simulink model "voltage_test"  (R2026a)
settings: Solver=VariableStepAuto  StopTime=inf
settings Model: Creator=user  LastModifiedBy=user

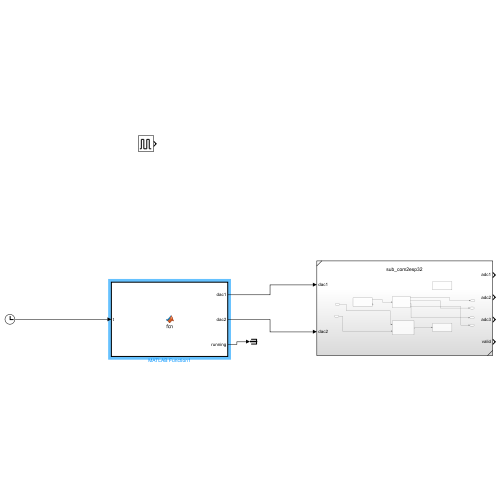
[thumbnail: Simulink's stored preview of the top-level diagram]
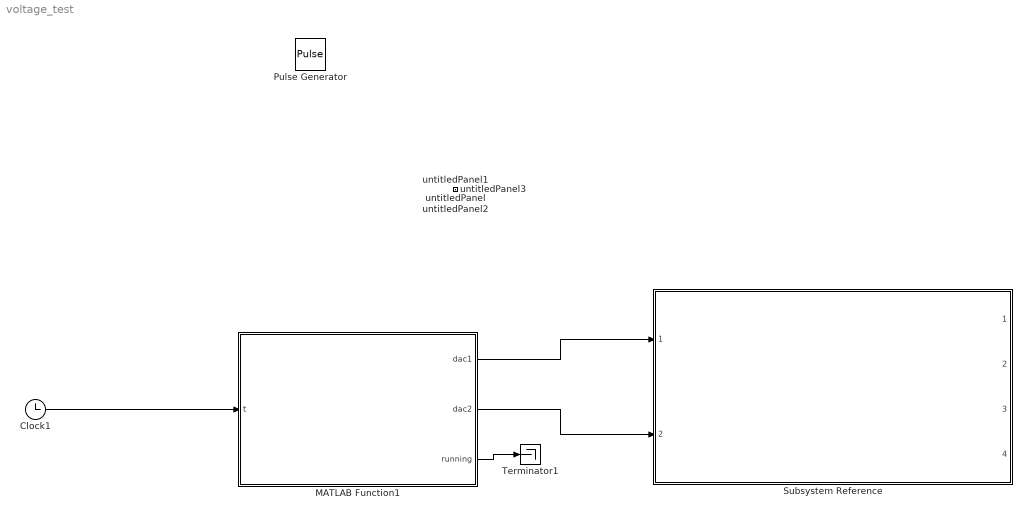
== system voltage_test ==
  Clock1 : Clock
  MATLAB Function1 : MATLAB Function  TreatAsAtomicUnit=on
  Pulse Generator : DiscretePulseGenerator  PulseType=Time based  Period=12  PulseWidth=20
  Subsystem Reference : Subsystem  ReferencedSubsystem=sub_com2esp32
  Terminator1 : Terminator
  untitledPanel : Subsystem  Tag=HiddenForWebPanel  IsWebBlockPanel=on
  untitledPanel1 : Subsystem  Tag=HiddenForWebPanel  IsWebBlockPanel=on
  untitledPanel2 : Subsystem  Tag=HiddenForWebPanel  IsWebBlockPanel=on
  untitledPanel3 : Subsystem  Tag=HiddenForWebPanel  IsWebBlockPanel=on
  wires:
  MATLAB Function1/1(dac1) -> Subsystem Reference/1
  MATLAB Function1/3(running) -> Terminator1/1
  MATLAB Function1/2(dac2) -> Subsystem Reference/2
  Clock1/1 -> MATLAB Function1/1(t)

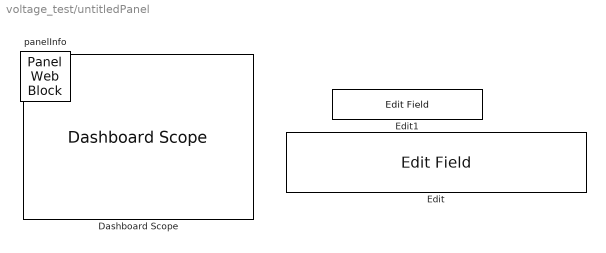
== system voltage_test/untitledPanel ==
  Dashboard Scope : DashboardScope  Tag=HiddenForWebPanel  PanelInfo="{\"height\":195,\"left\":22,\"panelId\":\"panelId-0a8f6d05-5e0e-4052-8464-4cdde78ccbfe\",\"top\":22,\"type\":\"panelChild\",\"version\":\"2019b\",\"width\":271,\"zIndex\":1500002}"  FontColor=[0.0, 0.0, 0.0]
  Edit : EditField  Tag=HiddenForWebPanel  PanelInfo="{\"height\":25,\"left\":322,\"panelId\":\"panelId-0a8f6d05-5e0e-4052-8464-4cdde78ccbfe\",\"top\":100,\"type\":\"panelChild\",\"version\":\"2019b\",\"width\":181,\"zIndex\":1500006}"  LabelPosition=Hide  ShowInitialText=on  Alignment=Center
  Edit1 : EditField  Tag=HiddenForWebPanel  PanelInfo="{\"height\":30,\"left\":327,\"panelId\":\"panelId-0a8f6d05-5e0e-4052-8464-4cdde78ccbfe\",\"top\":53,\"type\":\"panelChild\",\"version\":\"2019b\",\"width\":150,\"zIndex\":1500004}"  LabelPosition=Hide  ShowInitialText=on  Alignment=Center
  panelInfo : PanelWebBlock  Tag=HiddenForWebPanel  PanelInfo="{\"compacted\":false,\"height\":362,\"isActiveTab\":false,\"left\":183,\"name\":\"Panel\",\"panelId\":\"panelId-0a8f6d05-5e0e-4052-8464-4cdde78ccbfe\",\"popoutData\":{\"height\":495,\"left\":546,\"maximized\":false,\"top\":827,\"width\":618},\"popoutMode\":\"windowHidden\",\"tabIndex\":0,\"tabbedSetId\":\"tabbedSet4972758365\",\"top\":737,\"type\":\"panel\",\"version\":\"2019b\",\"visible\":false,\"width\":602,\"zIndex\":1500002}"  PanelSnapshot=<binary blob, 20028 chars, not shown>

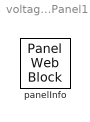
== system voltage_test/untitledPanel1 ==
  panelInfo : PanelWebBlock  Tag=HiddenForWebPanel  PanelInfo="{\"compacted\":false,\"height\":362,\"isActiveTab\":true,\"left\":183,\"name\":\"Panel1\",\"panelId\":\"panelId-b2ee2f41-7720-49f1-b51a-3062c351f597\",\"popoutData\":{\"height\":495,\"left\":546,\"maximized\":false,\"top\":827,\"width\":618},\"popoutMode\":\"windowHidden\",\"tabIndex\":1,\"tabbedSetId\":\"tabbedSet4972758365\",\"top\":737,\"type\":\"panel\",\"version\":\"2019b\",\"visible\":true,\"width\":602,\"zIndex\":1500004}"

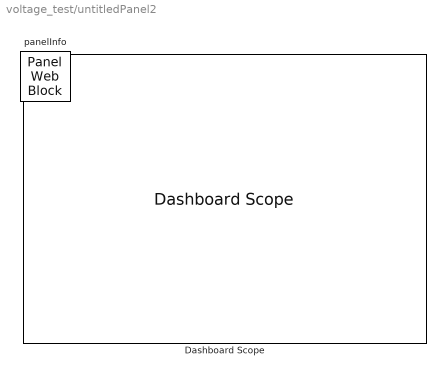
== system voltage_test/untitledPanel2 ==
  Dashboard Scope : DashboardScope  Tag=HiddenForWebPanel  PanelInfo="{\"height\":289,\"left\":18,\"panelId\":\"panelId-8ba459e9-7eb9-43d1-9a8b-2b7bff5a2d5c\",\"top\":18,\"type\":\"panelChild\",\"version\":\"2019b\",\"width\":403,\"zIndex\":1500002}"  FontColor=[0.0, 0.0, 0.0]
  panelInfo : PanelWebBlock  Tag=HiddenForWebPanel  PanelInfo="{\"compacted\":false,\"height\":329,\"isActiveTab\":true,\"left\":1320,\"name\":\"Panel2\",\"panelId\":\"panelId-8ba459e9-7eb9-43d1-9a8b-2b7bff5a2d5c\",\"popoutData\":{\"height\":440,\"left\":1683,\"maximized\":false,\"top\":822,\"width\":459},\"popoutMode\":\"windowHidden\",\"tabIndex\":0,\"tabbedSetId\":\"tabbedSet1724704130\",\"top\":710,\"type\":\"panel\",\"version\":\"2019b\",\"visible\":true,\"width\":443,\"zIndex\":1500006}"  PanelSnapshot=<binary blob, 75208 chars, not shown>

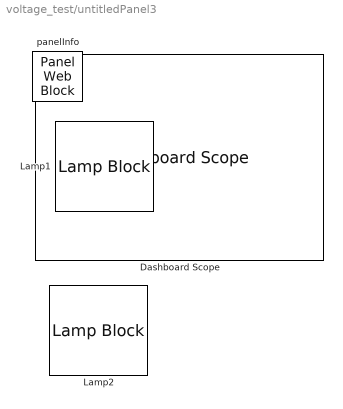
== system voltage_test/untitledPanel3 ==
  Dashboard Scope : DashboardScope  Tag=HiddenForWebPanel  PanelInfo="{\"height\":364,\"left\":211,\"panelId\":\"panelId-037cc253-1a0e-430c-bfc3-d197bdfa8fb6\",\"top\":20,\"type\":\"panelChild\",\"version\":\"2019b\",\"width\":531,\"zIndex\":1500002}"  FontColor=[0.0, 0.0, 0.0]
  Lamp1 : LampBlock  Tag=HiddenForWebPanel  PanelInfo="{\"height\":82,\"left\":28,\"panelId\":\"panelId-037cc253-1a0e-430c-bfc3-d197bdfa8fb6\",\"top\":79,\"type\":\"panelChild\",\"version\":\"2019b\",\"width\":89,\"zIndex\":1500004}"  LabelPosition=Hide  DefaultColor=[192.0, 192.0, 192.0]
  Lamp2 : LampBlock  Tag=HiddenForWebPanel  PanelInfo="{\"height\":82,\"left\":29,\"panelId\":\"panelId-037cc253-1a0e-430c-bfc3-d197bdfa8fb6\",\"top\":226,\"type\":\"panelChild\",\"version\":\"2019b\",\"width\":89,\"zIndex\":1500006}"  LabelPosition=Hide  DefaultColor=[192.0, 192.0, 192.0]
  panelInfo : PanelWebBlock  Tag=HiddenForWebPanel  PanelInfo="{\"compacted\":false,\"height\":411,\"isActiveTab\":true,\"labels\":{\"label0415151059\":{\"deleted\":false,\"left\":29,\"settings\":{\"backgroundColor\":\"rgba(0, 0, 0, 0)\",\"bold\":true,\"font\":\"Arial\",\"fontColor\":\"black\",\"fontSize\":1.09,\"italicized\":false,\"underlined\":false},\"text\":\"Pump\",\"top\":54},\"label6487320007\":{\"deleted\":false,\"left\":27,\"settings\":{\"backgroundColor\":\"rgba(0, 0, 0, 0)\",\"bold\":true,\"font\":\"Arial\",\"fontColor\":\"black\",\"fontSize\":1,\"italicized\":false,\"underlined\":false},\"text\":\"Calibration finished\",\"top\":201}},\"left\":207,\"name\":\"Panel3\",\"panelId\":\"panelId-037cc253-1a0e-430c-bfc3-d197bdfa8fb6\",\"tabIndex\":0,\"tabbedSetId\":\"tabbedSet3591606152\",\"top\":31,\"type\":\"panel\",\"version\":\"2019b\",\"visible\":true,\"width\":760,\"zIndex\":1500008}"  PanelSnapshot=<binary blob, 133644 chars, not shown>

== matlab function voltage_test/MATLAB Function1 ==
  data: t input; dac1 output; dac2 output; running output

function [dac1,dac2,running] = fcn(t)

dac1 = 250;
dac2 = 250;
running = 1;

end
